simulink model "system_sim_test3"  (R2015a)
settings: Solver=ode45  StartTime=0.0  StopTime=100  RelTol=1e-3
values from neighbouring files (symbols this model uses):
  area = 2    [run_sim_test2.m]    (also in run_sim_test4.m; run_sim_v2_test.m)
  Cd = 1    [run_sim_test2.m]    (also in run_sim_test4.m; run_sim_v2_test.m)
  m = 150    [run_sim_test2.m]    (also in run_sim_test4.m; run_sim_v2_test.m)
  rho_air = 1.225    [run_sim.m]    (also in run_sim_test.m; run_sim_test2.m; run_sim_test4.m; run_sim_v2_test.m)
settings Model: Creator=marco  LastModifiedBy=marco

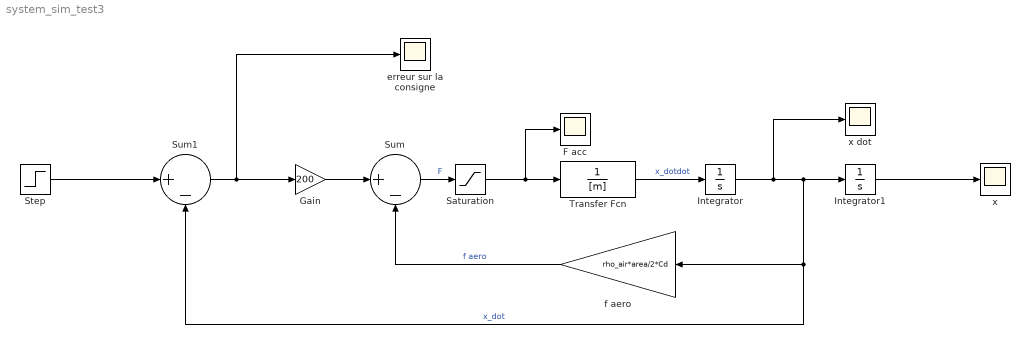
== system system_sim_test3 ==
  F acc : Scope
      settings: SaveName=ScopeData7
  Gain : Gain  Gain=200
  Integrator : Integrator
  Integrator1 : Integrator
  Saturation : Saturate  UpperLimit=150  LowerLimit=-150
  Step : Step  Time=0  After=4.16  SampleTime=0
  Sum : Sum  Inputs=|+-
  Sum1 : Sum  Inputs=|+-
  Transfer Fcn : TransferFcn  Denominator=[m]
  erreur sur la consigne : Scope
      settings: SaveName=ScopeData12
  f aero : Gain  Gain=rho_air*area/2*Cd
  x : Scope
  x dot : Scope
      settings: SaveName=ScopeData13
  wires:
  Sum/1 -> Saturation/1  "F"
  Transfer Fcn/1 -> Integrator/1  "x_dotdot"
  Integrator/1 -> x dot/1, Sum1/2, f aero/1, Integrator1/1  "x_dot"
  f aero/1 -> Sum/2  "f aero"
  Integrator1/1 -> x/1
  Step/1 -> Sum1/1
  Sum1/1 -> erreur sur la consigne/1, Gain/1
  Gain/1 -> Sum/1
  Saturation/1 -> F acc/1, Transfer Fcn/1
